simulink model "bObserver"  (R2020a)
settings: Solver=VariableStepAuto  StartTime=0.0  StopTime=1.5  FixedStep=0.0005  EnableMultiTasking=on
InitFcn:
  | kp=0.01;
  | ki=0.01;
  | 
  | k=2;
  | em=100000000;
  | GE=1/em;
  | GU=k*ki/GE;
  | GCE=k*kp/GU;
model workspace (MAT data in the model file):
  time = 0.8
values from neighbouring files (symbols this model uses):
  A1 = obj.boostConverter.A1    [BoostController.m]    (also in BoostConverter.m = [-obj.R/obj.L 0;0 -1/(obj.Ro*obj.C)]; BuckBoostConverter.m = [-obj.R/obj.L 0;0 -1/(obj.Ro*obj.C)]; obsmc.m = Asigma{1,1}; workspace_atual.mat = [-16.4  0; 0  -3.50877192982])
  A2 = obj.boostConverter.A2    [BoostController.m]    (also in BoostConverter.m = [-obj.R/obj.L -1/obj.L;1/obj.C -1/(obj.Ro*obj.C)]; BuckBoostConverter.m = [-obj.R/obj.L 1/obj.L;-1/obj.C -1/(obj.Ro*obj.C)]; obsmc.m = Asigma{1,2}; workspace_atual.mat = [-16.4  -200; 350.877192982  -3.50877192982])
  AlarmDeadTime = 0.50    (= 0.5)    [BoostFaultSimulation.m]    (also in workspace_atual.mat; workspace_certo.mat)
  B1 = obj.boostConverter.B1    [BoostController.m]    (also in BoostConverter.m = [1/obj.L;0]; BuckBoostConverter.m = [1/obj.L;0]; obsmc.m = Bsigma{1,1}; workspace_atual.mat = [200 0])
  B1f = [200 0]    [workspace_atual.mat]    (also in workspace_certo.mat)
  B2 = obj.boostConverter.B2    [BoostController.m]    (also in BoostConverter.m = obj.B1; obsmc.m = Bsigma{1,2}; workspace_atual.mat = [200 0]; workspace_certo.mat = [200 0])
  B2f = [200 0]    [workspace_atual.mat]    (also in workspace_certo.mat)
  boost_Amatrices = cat(3,obj.A1,obj.A2)    [BoostConverter.m]    (also in BuckBoostConverter.m; boostResults2Latex.m = boost.A_matrices(); workspace_atual.mat = [-16.4 0 0 -3.50877192982 -16.4 350.877192982 -200 -3.508771; workspace_certo.mat = [-16.4 0 0 -3.50877192982 -16.4 350.877192982 -200 -3.508771)
  boost_parameters = [obj.Ro,obj.R,obj.L,obj.C,obj.u]'    [BoostConverter.m]    (also in BuckBoostConverter.m; boostResults2Latex.m = boost.parameters(); workspace_atual.mat = [100 0.082 0.005 0.00285 190]; workspace_certo.mat = [100 0.082 0.005 0.00285 190])
  C = 1e-3    (= 0.001)    [boostResults2Latex.m]
  CiL = [0 1]    [workspace_atual.mat]    (also in workspace_certo.mat)
  Cmatrix = [1  0; 0  1]    [workspace_atual.mat]    (also in workspace_certo.mat)
  CVc = [1 0]    [workspace_atual.mat]    (also in workspace_certo.mat)
  D1 = [1  0; 0  1]    [workspace_atual.mat]    (also in workspace_certo.mat)
  F_11 = -16.4    [workspace_atual.mat]    (also in workspace_certo.mat)
  F_12 = -4812476.87956    [workspace_atual.mat]    (also in workspace_certo.mat)
  F_21 = -3.50877192982    [workspace_atual.mat]    (also in workspace_certo.mat)
  F_22 = -2.00703596657    [workspace_atual.mat]    (also in workspace_certo.mat)
  FaultClass = 0    [BoostFaultSimulation.m]    (also in workspace_atual.mat = 1; workspace_certo.mat = 1)
  H_1 = 13715.5123667    [workspace_atual.mat]    (also in workspace_certo.mat)
  iLFaultSwitch = 0    [BoostFaultSimulation.m]    (also in workspace_atual.mat; workspace_certo.mat)
  iLFaultTime = 1.70    (= 1.7)    [BoostFaultSimulation.m]    (also in workspace_atual.mat; workspace_certo.mat)
  iLGainFaultFactor = 15    [BoostFaultSimulation.m]    (also in workspace_atual.mat; workspace_certo.mat)
  iLNoiseFaultSwitch = 0    [BoostFaultSimulation.m]    (also in workspace_atual.mat; workspace_certo.mat)
  iLNoiseTime = 1.70    (= 1.7)    [BoostFaultSimulation.m]    (also in workspace_atual.mat; workspace_certo.mat)
  Jth = 2000    [workspace_atual.mat]    (also in workspace_certo.mat)
  L = 1e-3    (= 0.001)    [boostResults2Latex.m]    (also in obsmc.m = sdpvar(3,1,'full'))
  L_11 = -176809.798019    [workspace_atual.mat]    (also in workspace_certo.mat)
  L_12 = -66005538231.6    [workspace_atual.mat]    (also in workspace_certo.mat)
  L_21 = 0.0967961040176    [workspace_atual.mat]    (also in workspace_certo.mat)
  L_22 = 350.985265141    [workspace_atual.mat]    (also in workspace_certo.mat)
  LoadAddSignalSwitch = 1    [BoostFaultSimulation.m]    (also in workspace_atual.mat; workspace_certo.mat)
  LoadAddSwitch = 0    [BoostFaultSimulation.m]    (also in workspace_atual.mat; workspace_certo.mat)
  LoadAddTime = 0.90    (= 0.9)    [BoostFaultSimulation.m]    (also in workspace_atual.mat; workspace_certo.mat)
  LoadRemoveSignalSwitch = 1    [BoostFaultSimulation.m]    (also in workspace_atual.mat; workspace_certo.mat)
  LoadRemoveSwitch = 0    [BoostFaultSimulation.m]    (also in workspace_atual.mat; workspace_certo.mat)
  LoadRemoveTime = 0.90    (= 0.9)    [BoostFaultSimulation.m]    (also in workspace_atual.mat; workspace_certo.mat)
  LobsiL = [1737913.15707 66180.0912281]    [workspace_atual.mat]    (also in workspace_certo.mat)
  LobsVc = [61200 1]    [workspace_atual.mat]    (also in workspace_certo.mat)
  ObsEp = 70    [workspace_atual.mat]    (also in workspace_certo.mat)
  P = value(P)    [BoostController.m]    (also in boostResults2Latex.m = boost.calculateP(); obsmc.m = blkdiag(1/deltaAtilde(1,2),-1/deltaAtilde(2,1),1); workspace_atual.mat = [0.00235275094895  5.25738510027e-05; 5.25738510027e-05  0.0; workspace_certo.mat = [0.00235275094893  5.25738512446e-05; 5.25738512446e-05  0.0)
  Q_1 = [13715.5123667  1; 1  0]    [workspace_atual.mat]    (also in workspace_certo.mat)
  Q_2 = [1  0; 0.00750867981628  1]    [workspace_atual.mat]    (also in workspace_certo.mat)
  R = 0.1    [boostResults2Latex.m]    (also in workspace_atual.mat = 0.082; workspace_certo.mat = 0.082)
  ReconfigSwitch = 0    [BoostFaultSimulation.m]    (also in workspace_atual.mat; workspace_certo.mat)
  ReconfigTime = 1.707    [BoostFaultSimulation.m]    (also in workspace_atual.mat; workspace_certo.mat)
  rho = 5    [workspace_atual.mat]    (also in workspace_certo.mat)
  RMSfrequency = 47.61    [BoostFaultSimulation.m]    (also in workspace_atual.mat; workspace_certo.mat)
  Ro = 100    [BoostFaultSimulation.m]    (also in boostResults2Latex.m = 10; workspace_atual.mat; workspace_certo.mat)
  Smep = 80    [workspace_atual.mat]    (also in workspace_certo.mat)
  SourceAddSignalSwitch = 1    [BoostFaultSimulation.m]    (also in workspace_atual.mat; workspace_certo.mat)
  SourceAddSwitch = 0    [BoostFaultSimulation.m]    (also in workspace_atual.mat; workspace_certo.mat)
  SourceAddTime = 0.90    (= 0.9)    [BoostFaultSimulation.m]    (also in workspace_atual.mat; workspace_certo.mat)
  SourceAddVoltage = obj.SourceAddFactor*obj.u    [BoostFaultSimulation.m]    (also in workspace_atual.mat = 19; workspace_certo.mat = 19)
  SourceRemoveSignalSwitch = 1    [BoostFaultSimulation.m]    (also in workspace_atual.mat; workspace_certo.mat)
  SourceRemoveSwitch = 0    [BoostFaultSimulation.m]    (also in workspace_atual.mat; workspace_certo.mat)
  SourceRemoveTime = 0.90    (= 0.9)    [BoostFaultSimulation.m]    (also in workspace_atual.mat; workspace_certo.mat)
  SourceRemoveVoltage = obj.SourceRemoveFactor*obj.u    [BoostFaultSimulation.m]    (also in workspace_atual.mat = 19; workspace_certo.mat = 19)
  T_1 = [1 -13715.5123667]    [workspace_atual.mat]    (also in workspace_certo.mat)
  T_2 = [-0.00750867981628 1]    [workspace_atual.mat]    (also in workspace_certo.mat)
  ueq = 0.5    [workspace_atual.mat]    (also in workspace_certo.mat)
  uf = 190    [workspace_atual.mat]    (also in workspace_certo.mat)
  VcFaultSwitch = 0    [BoostFaultSimulation.m]    (also in workspace_atual.mat; workspace_certo.mat)
  VcFaultTime = 1.70    (= 1.7)    [BoostFaultSimulation.m]    (also in workspace_atual.mat; workspace_certo.mat)
  VcGainFaultFactor = 15    [BoostFaultSimulation.m]    (also in workspace_atual.mat; workspace_certo.mat)
  VcNoiseFaultSwitch = 0    [BoostFaultSimulation.m]    (also in workspace_atual.mat; workspace_certo.mat)
  VcNoiseTime = 1.70    (= 1.7)    [BoostFaultSimulation.m]    (also in workspace_atual.mat; workspace_certo.mat)
  ve = 380    [BoostFaultSimulation.m]    (also in boostResults2Latex.m = 100; workspace_atual.mat; workspace_certo.mat)
  x_e = [ie;ve]    [BoostConverter.m]    (also in BuckBoostConverter.m)
  xe = obj.boostConverter.equilibriumstate(ve)    [BoostController.m]    (also in workspace_atual.mat = [7.62509288104 380]; workspace_certo.mat = [7.62509288104 380])
undefined symbols (not defined in the file or in its folder): Atilde1, Atilde2, B1u, Ctilde1, Dtilde1, Dtilde2, F, F1, G, G1, MAXnet, MINnet
libraries: neural x36, powerlib x34, dspstat3 x11, PhdLibrary x10, simulink x7, dspmtrx3 x6, powerlib_meascontrol x4, dspmathops x4
(part 1 of 6)
settings Model: SimulationMode=accelerator  Creator=d13go  LastModifiedBy=vitor
settings SolverCC: MaxConsecutiveZCs=10000  ZeroCrossAlgorithm=Adaptive  DecoupledContinuousIntegration=on  MinimalZcImpactIntegration=on
settings DataIOCC: SaveFinalState=on  SaveState=on  LoggingToFile=on
settings OptimizationCC: DefaultParameterBehavior=Inlined  UseDivisionForNetSlopeComputation=on  GainParamInheritBuiltInType=on  UseFloatMulNetSlope=on  InlineInvariantSignals=on  EfficientFloat2IntCast=on  LifeSpan=1
settings DebuggingCC: ReadBeforeWriteMsg=DisableAll  WriteAfterWriteMsg=DisableAll  WriteAfterReadMsg=DisableAll  AlgebraicLoopMsg=error  MaxConsecutiveZCsMsg=warning  MaskedZcDiagnostic=none  IgnoredZcDiagnostic=none  MultiTaskDSMMsg=none  SFUnexpectedBacktrackingDiag=warning  SFNoUnconditionalDefaultTransitionDiag=warning  ArithmeticOperatorsInVariantConditions=warning
settings HardwareCC: ProdLongLongMode=on
settings ModelReferenceCC: UpdateModelReferenceTargets=IfOutOfDate
settings SFSimCC: SFSimEcho=off  SimUseLocalCustomCode=off  MATLABDynamicMemAlloc=off  CustomCodeUndefinedFunction=UseInterfaceOnly
settings RTWCC: GenerateReport=on  RTWUseLocalCustomCode=off  LaunchReport=on
settings CodeAppCC: ForceParamTrailComments=on
settings GRTTargetCC: TargetLangStandard=C89/C90 (ANSI)  CombineSignalStateStructs=on  MatFileLogging=off  SupportVariableSizeSignals=on
settings ConfigComp: CovMetricSettings=dw  CovHtmlReporting=on  CovSaveCumulativeToWorkspaceVar=on  CovSaveSingleToWorkspaceVar=on  CovExternalEMLEnable=off
settings SimscapeCC: SimscapeNormalizeSystem=off

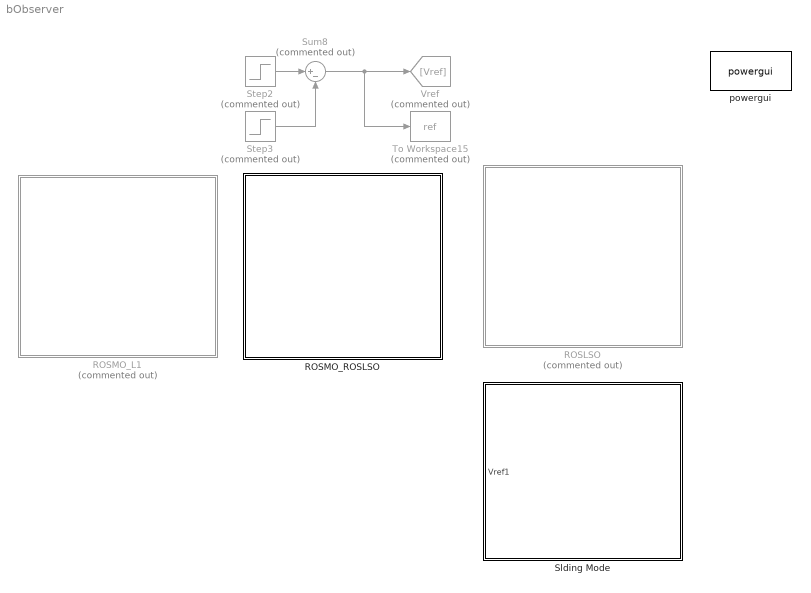
== system bObserver ==
  ROSLSO : Subsystem  Commented=on
  ROSMO_L1 : Subsystem  Commented=on
  ROSMO_ROSLSO : Subsystem
  Slding Mode : Subsystem
  Step2 : Step  Commented=on  Time=0  After=100  SampleTime=0
  Step3 : Step  Commented=on  Time=0.4  After=20  SampleTime=0
  Sum8 : Sum  Commented=on  Inputs=|+-
  To Workspace15 : ToWorkspace  Commented=on  VariableName=ref  SampleTime=-1
  Vref : Goto  Commented=on  GotoTag=Vref
  powergui : powerlib/powergui  Priority=1  SimulationMode=Discrete  SampleTime=50e-6  frequency=60  Iterations=50  frequencyindice=0  Pbase=100e6  ErrMax=1e-4  UnitsV=kV  UnitsW=MW  buscounter=0  FunctionMessages=off  echomessages=off  EnableUseOfTLC=off  CurrentSourceSwitches=off  DisableSnubberDevices=off  DisableRonSwitches=off  DisableVfSwitches=off  DisplayEquations=off  AutomaticDiscreteSolvers=off  SolverType=Tustin/Backward Euler (TBE)  Interpol=off  ExternalGateDelay=off  methode=off  Ts=100  x0status=blocks  SPID=on  SwTol=0  HookPort=off  NonlinearTolerance=1e-4  nMaxIteration=100  ContinueOnMaxIteration=off  RestoreLinks=warning  ResistiveCurrentMeasurement=off  Frange=[0:2:500]  Ylog=off  Xlog=on  ShowGrid=off  save=off  variable=ZData  structure=0  ZoomFFT=off  StartTime=0.0  cycles=1  DisplayStyle=1  fundamental=60  FreqAxis=off  MaxFrequency=1000  frequencyindicesteady=1  RmsSteady=1  display=off
  wires:
  Step2/1 -> Sum8/1
  Step3/1 -> Sum8/2
  Sum8/1 -> To Workspace15/1, Vref/1

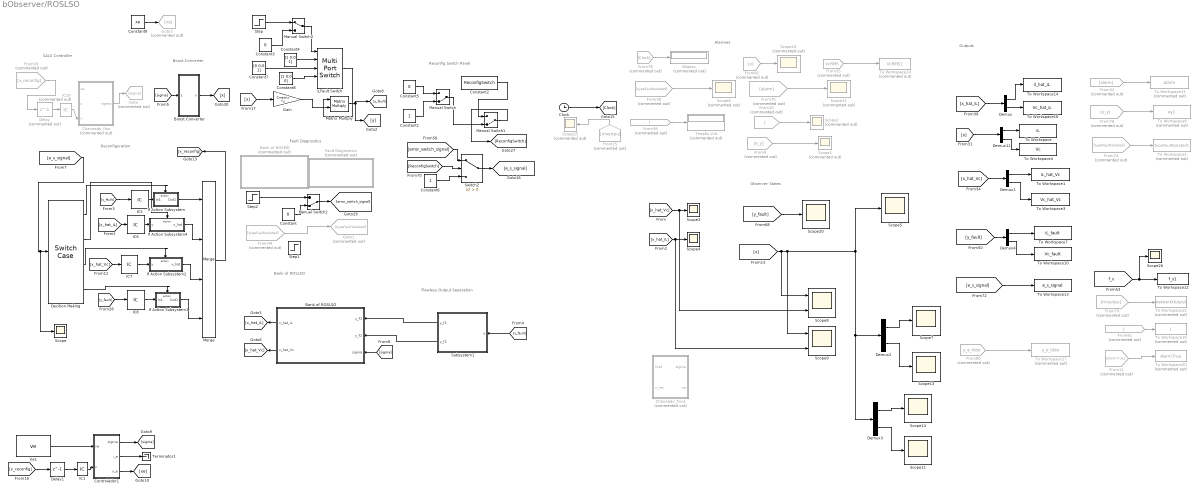
== system bObserver/ROSLSO ==
  note: Fault Diagnostics
  note: Bank of ROSLSO
  note: Reconfiguration
  note: SALS Controller
  note: Boost Converter
  note: Reconfig Switch Panel
  note: Observer States
  note: Outputs
  note: Alarmes
  note: Flawless Output Separation
  Bank of ROSLSO : Subsystem
  Bank of ROSMO : Subsystem  Commented=on
  Boost Converter : Subsystem
  Chaveado_fixo : Subsystem  Commented=on  mask(Switched linear affine Controler){A1=0, A2=0, B1=0, B2=0, P=0}
      mask prompts: A1 "System matrix 1:"; A2 "System matrix 2:"; B1 "Input matrix 1:"; B2 "Input matrix 2:"; P "Gain matrix:"
      mask help: Controller to generate a switching law according to the equilibrium point xe
  Chaveado_fixo1 : Subsystem  Commented=on
  Clock : Clock
  Constant : Constant  Value=0
  Constant1 : Constant
  Constant2 : Constant  Value=ReconfigSwitch
  Constant3 : Constant  Value=0
  Constant4 : Constant  Value=[1 0;0 1]  VectorParams1D=off
  Constant5 : Constant  Value=0
  Constant6 : Constant
  Constant7 : Constant  Value=[0 0;0 1]  VectorParams1D=off
  Constant8 : Constant  Value=[1 0;0 0]  VectorParams1D=off
  Constant9 : Constant  Value=xe
  Controlador1 : Subsystem
  Decition Making : SwitchCase  CaseConditions={[0],[1],[2]}
  Delay : Delay  Commented=on  DelayLength=1
  Delay1 : Delay  DelayLength=1
  Demux{,1..4,11} (6 alike) : Demux  Outputs=2
  Display : Display  Commented=on
  Fault Diagnostics : Subsystem  Commented=on
  From10 : From  Commented=on  GotoTag=J  TagVisibility=global
  From11 : From  Commented=on  GotoTag=alarmTrue
  From15 : From  Commented=on  GotoTag=nnoutpu
  From32 : From  Commented=on  GotoTag=alarm
  From33 : From  Commented=on  GotoTag=x_reconfig
  From35 : From  Commented=on  GotoTag=VcRMS  TagVisibility=global
  From36 : From  Commented=on  GotoTag=J  TagVisibility=global
  From38 : From  Commented=on  GotoTag=typeFaultIsolated
  From44 : From  Commented=on  GotoTag=typeFaultIsolated
  From74 : From  Commented=on  GotoTag=typeFaultIsolated
  From75 : From  Commented=on  GotoTag=alarm
  From76 : From  Commented=on  GotoTag=e_y
  From78 : From  Commented=on  GotoTag=Clock
  From79 : From  Commented=on  GotoTag=nnoutpu
  From80 : From  Commented=on  GotoTag=y_e_tilde  TagVisibility=global
  From81 : From  Commented=on  GotoTag=J  TagVisibility=global
  From82 : From  Commented=on  GotoTag=v
  From9 : From  Commented=on  GotoTag=e_y
  Gain : Gain  Gain=Cmatrix  Multiplication=Matrix(K*u)
  Goto : Goto  Commented=on  GotoTag=sigma
  Goto1 : Goto  Commented=on  GotoTag=typeFaultIsolated
  Goto3 : Goto  Commented=on  GotoTag=xe
  IC{1,5..8} (5 alike) : InitialCondition  Value=[0;0]
  IC10 : InitialCondition  Commented=on  Value=[0;0]
  If Action Subsystem : Subsystem  TreatAsAtomicUnit=on
  If Action Subsystem1 : Subsystem  TreatAsAtomicUnit=on
  If Action Subsystem2 : Subsystem  TreatAsAtomicUnit=on
  If Action Subsystem4 : Subsystem  TreatAsAtomicUnit=on
  Manual Switch : ManualSwitch  CurrentSetting=0
  Manual Switch1 : ManualSwitch  CurrentSetting=0
  Manual Switch2 : ManualSwitch  CurrentSetting=0
  Manual Switch3 : ManualSwitch
  Matrix Multiply : Product  Multiplication=Matrix(*)
  Merge : Merge  Inputs=4
  Scope{,3..5,7,11,13..14,20,26} (10 alike) : Scope
  Scope{1..2,6,10,12,25} (6 alike) : Scope  Commented=on
  Scope8 : Scope  NumInputPorts=2
  Scope9 : Scope  NumInputPorts=2
  Step : Step  Time=0.5  After=2  SampleTime=0
  Step1 : Step  Time=ReconfigTime  Before=1  After=FaultClass  SampleTime=0
  Step2 : Step  Time=0.510  After=2  SampleTime=0
  Subsystem1 : Subsystem
  Switch2 : Switch  Criteria=u2 > Threshold
  Tensão Vc6 : Display  Commented=on
  Terminator1 : Terminator
  To Workspace : ToWorkspace  VariableName=iL  SaveFormat=Timeseries  SampleTime=-1
  To Workspace1 : ToWorkspace  VariableName=iL_hat_Vc  SaveFormat=Timeseries  SampleTime=-1
  To Workspace10 : ToWorkspace  VariableName=Vc_fault  SaveFormat=Timeseries  SampleTime=-1
  To Workspace11 : ToWorkspace  Commented=on  VariableName=Alarm  SaveFormat=Timeseries  SampleTime=-1
  To Workspace12 : ToWorkspace  VariableName=f_s1  SaveFormat=Timeseries  SampleTime=-1
  To Workspace13 : ToWorkspace  VariableName=e_s_signal  SaveFormat=Timeseries  SampleTime=-1
  To Workspace14 : ToWorkspace  VariableName=il_hat_iL  SaveFormat=Timeseries  SampleTime=-1
  To Workspace15 : ToWorkspace  Commented=on  VariableName=networkOutput  SaveFormat=Timeseries  SampleTime=-1
  To Workspace16 : ToWorkspace  VariableName=Vc_hat_iL  SaveFormat=Timeseries  SampleTime=-1
  To Workspace17 : ToWorkspace  Commented=on  VariableName=y_e_tilde  SaveFormat=Timeseries  SampleTime=-1
  To Workspace19 : ToWorkspace  Commented=on  VariableName=J  SaveFormat=Timeseries  SampleTime=-1
  To Workspace2 : ToWorkspace  Commented=on  VariableName=typeFaultIsolated1  SaveFormat=Timeseries  SampleTime=-1
  To Workspace20 : ToWorkspace  Commented=on  VariableName=AlarmTrue  SaveFormat=Timeseries  SampleTime=-1
  To Workspace24 : ToWorkspace  Commented=on  VariableName=VcRMS1  SaveFormat=Timeseries  SampleTime=-1
  To Workspace3 : ToWorkspace  VariableName=Vc_hat_Vc  SaveFormat=Timeseries  SampleTime=-1
  To Workspace4 : ToWorkspace  VariableName=Vc  SaveFormat=Timeseries  SampleTime=-1
  To Workspace7 : ToWorkspace  VariableName=iL_fault  SaveFormat=Timeseries  SampleTime=-1
  To Workspace8 : ToWorkspace  Commented=on  VariableName=ey1  SaveFormat=Timeseries  SampleTime=-1
  Ve1 : Constant  Value=ve
  iLFault Switch : MultiPortSwitch  DataPortOrder=Zero-based contiguous  DataPortForDefault=Additional data port  zeroidx=on
  wires:
  From9/1 -> Scope1/1
  From10/1 -> Scope2/1
  Manual Switch2/1 -> [error_switch_signal]
  Decition Making/1 -> If Action Subsystem/Action
  If Action Subsystem/1(Out1) -> Merge/1
  Decition Making/3 -> If Action Subsystem2/Action
  Clock/1 -> [Clock]
  [ReconfigSwitch] -> Switch2/2
  Manual Switch/1 -> Manual Switch1/2
  Constant1/1 -> Manual Switch/2
  Constant2/1 -> Manual Switch1/1
  Constant5/1 -> Manual Switch/1
  Constant6/1 -> Switch2/3
  Manual Switch1/1 -> [ReconfigSwitch]
  [error_switch_signal] -> Switch2/1
  Decition Making/2 -> If Action Subsystem4/Action
  [y_fault] -> IC8/1
  [x_hat_iL] -> Scope9/2, Scope4/1
  [sigma] -> Boost Converter/1(sigma)
  [x_hat_iL] -> Demux/1
  Demux/1 -> To Workspace14/1
  Demux1/2 -> To Workspace3/1
  From36/1 -> Tensão Vc6/1
  [y_fault] -> Demux4/1
  Demux4/2 -> To Workspace10/1
  From38/1 -> Scope6/1
  From75/1 -> Scope12/1
  From76/1 -> To Workspace8/1
  [f_s] -> Scope26/1, To Workspace12/1
  [y_fault] -> Scope20/1
  From32/1 -> To Workspace11/1
  [e_s_signal] -> To Workspace13/1
  Demux1/1 -> To Workspace1/1
  From74/1 -> To Workspace2/1
  From78/1 -> Display/1
  Demux/2 -> To Workspace16/1
  Demux4/1 -> To Workspace7/1
  [x_hat_Vc] -> Demux1/1
  From79/1 -> To Workspace15/1
  From80/1 -> To Workspace17/1
  From81/1 -> To Workspace19/1
  From82/1 -> Scope10/1
  IC5/1 -> If Action Subsystem/1(In1)
  [y_fault] -> IC5/1
  IC7/1 -> If Action Subsystem2/1(y)
  [x_hat_Vc] -> IC7/1
  IC8/1 -> If Action Subsystem1/1(In1)
  From11/1 -> To Workspace20/1
  Decition Making/4 -> If Action Subsystem1/Action
  IC6/1 -> If Action Subsystem4/1(y)
  If Action Subsystem4/1(x_hat) -> Merge/2
  If Action Subsystem2/1(x_hat) -> Merge/3
  If Action Subsystem1/1(Out1) -> Merge/4
  Merge/1 -> [x_reconfig]
  From15/1 -> Scope25/1
  [x_hat_Vc] -> Scope8/2, Scope3/1
  From35/1 -> To Workspace24/1
  [x] -> Demux11/1
  Demux11/1 -> To Workspace/1
  Demux11/2 -> To Workspace4/1
  [x_hat_iL] -> IC6/1
  [y_fault] -> Subsystem1/1(y)
  Subsystem1/1(y_f1) -> Bank of ROSLSO/1(y_f1)
  Subsystem1/2(y_f2) -> Bank of ROSLSO/2(y_f2)
  [sigma] -> Bank of ROSLSO/3(sigma)
  Bank of ROSLSO/1(x_hat_iL) -> [x_hat_iL]
  Bank of ROSLSO/2(x_hat_Vc) -> [x_hat_Vc]
  [x] -> Scope8/1, Scope9/1, Scope5/1, Demux3/1, Demux2/1
  Switch2/1 -> [e_s_signal]
  IC10/1 -> Chaveado_fixo/3(x)
  Constant9/1 -> Goto3/1
  Chaveado_fixo/1(sigma) -> Goto/1
  [x] -> Gain/1
  Gain/1 -> Matrix Multiply/2
  Matrix Multiply/1 -> [y], [y_fault]
  Constant4/1 -> iLFault Switch/2
  Constant8/1 -> iLFault Switch/4
  Constant7/1 -> iLFault Switch/3
  iLFault Switch/1 -> Matrix Multiply/1
  Boost Converter/1(x) -> [x]
  [e_s_signal] -> Scope/1, Decition Making/1
  Delay/1 -> IC10/1
  From33/1 -> Delay/1
  Step2/1 -> Manual Switch2/1
  Controlador1/3(x_e) -> [xe]
  Controlador1/1(sigma) -> [sigma]
  Controlador1/2(i_e) -> Terminator1/1
  IC1/1 -> Controlador1/2(x)
  [x_reconfig] -> Delay1/1
  Delay1/1 -> IC1/1
  Ve1/1 -> Controlador1/1(ve)
  Demux2/1 -> Scope7/1
  Demux2/2 -> Scope13/1
  Demux3/2 -> Scope11/1
  Demux3/1 -> Scope14/1
  Step/1 -> Manual Switch3/1
  Manual Switch3/1 -> iLFault Switch/1
  Constant3/1 -> Manual Switch3/2
  Constant/1 -> Manual Switch2/2
  From44/1 -> Goto1/1

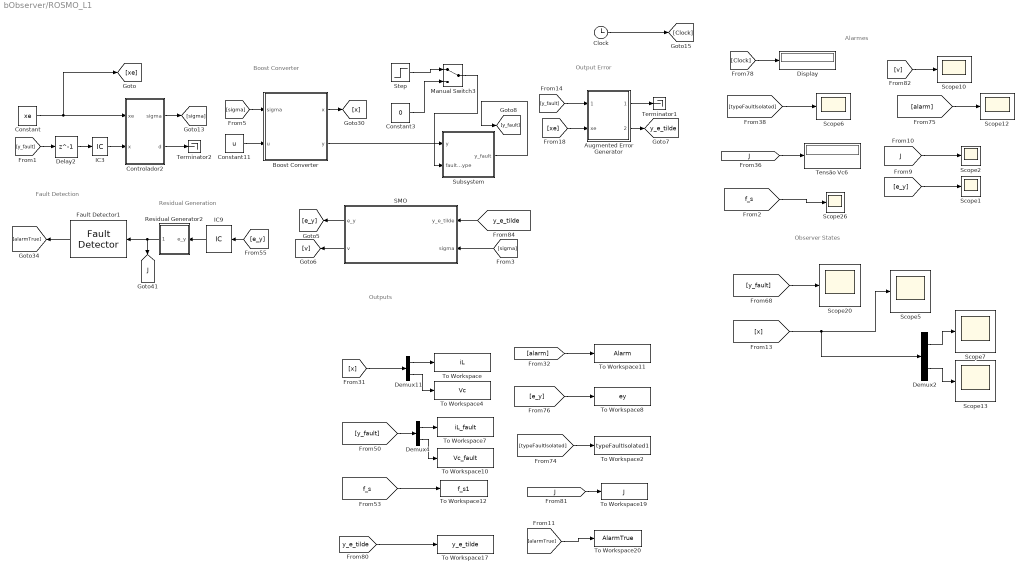
== system bObserver/ROSMO_L1 ==
  note: Boost Converter
  note: Observer States
  note: Outputs
  note: Alarmes
  note: Output Error
  note: Residual Generation
  note: Fault Detection
  Augmented Error Generator : Subsystem  mask{Cmatrix=Cmatrix, Ctilde1=Ctilde1}
      mask prompts: Cmatrix "Output Matrix"; Ctilde1 "Output matrix augmented:"
  Boost Converter : Subsystem  mask(Boots State-Space model){A1=A1, A2=A2, B1=B1, R=R, Ro=Ro, Cmatrix=Cmatrix}
      mask prompts: A1 "A1 matrix"; A2 "A2 matrix"; B1 "B matrix"; R "Resistance"; Ro "Output Resistance"; Cmatrix "Output Matrix"
      mask help: Boots State-Space model
      mask Display: disp('Boost')
  Clock : Clock
  Constant : Constant  Value=xe  VectorParams1D=off
  Constant11 : Constant  Value=u
  Constant3 : Constant  Value=0
  Controlador2 : Subsystem  mask(Sliding mode controller){KiVc=2.3, KVc=0.2, ueq=ueq, Smep=Smep, KiL=2, Freq=7000}
      mask prompts: KiVc "Integral voltage gain"; KVc "Voltage gain"; ueq "Equilibrium signal"; Smep "Surface limit layer"; KiL "Current gain"; Freq "Frequency"
      mask help: Sliding mode controller with integral for boost converter
  Delay2 : Delay  DelayLength=1
  Demux11 : Demux  Outputs=2
  Demux2 : Demux  Outputs=2
  Demux4 : Demux  Outputs=2
  Display : Display
  Fault Detector1 : PhdLibrary/Fault Detector  Jth=0
      settings: SourceProductName=Phd Diego
  IC3 : InitialCondition  Value=[0;0]
  IC9 : InitialCondition  Value=[0;0]
  Manual Switch3 : ManualSwitch
  Residual Generator2 : Subsystem  mask{RMSfrequency=RMSfrequency/10}
      mask prompts: RMSfrequency "Windows length:"
      mask help: RMS generator for two dimensios
  SMO : Subsystem  mask(Sliding mode observer){G=G1, F=F1, Atilde1=Atilde1, Atilde2=Atilde2, Dtilde1=Dtilde1, Dtilde2=Dtilde2, Ctilde1=Ctilde1, rho=rho}
      mask prompts: G "G matrix"; F "F matrix"; Atilde1 "A1 matrix augmented"; Atilde2 "A2 matrix augmented"; Dtilde1 "D1 matrix augmented"; Dtilde2 "D2 matrix augmented"; Ctilde1 "C1 matrix augmented"; rho "Sliding surface coefficient (rho)"
      mask help: Sligin mode observer for fault detection in switched affine linear systems
      mask Help: Enter the system matrices and the observer gains
      mask Display: disp('\dot{x} = Ax + b \\ y = Cx','texmode','on');
  Scope{1..2,5..7,10,12..13,20,26} (10 alike) : Scope
  Step : Step  Time=0.70  SampleTime=0
  Subsystem : Subsystem  mask(Step faults){iLfgain=20, Vcfgain=20}
      mask prompts: iLfgain "Current fault gain (A)"; Vcfgain "Voltage fault gain (V)"
      mask help: Configure a step fault
  Tensão Vc6 : Display
  Terminator1 : Terminator
  Terminator2 : Terminator
  To Workspace : ToWorkspace  VariableName=iL  SaveFormat=Timeseries  SampleTime=-1
  To Workspace10 : ToWorkspace  VariableName=Vc_fault  SaveFormat=Timeseries  SampleTime=-1
  To Workspace11 : ToWorkspace  VariableName=Alarm  SaveFormat=Timeseries  SampleTime=-1
  To Workspace12 : ToWorkspace  VariableName=f_s1  SaveFormat=Timeseries  SampleTime=-1
  To Workspace17 : ToWorkspace  VariableName=y_e_tilde  SaveFormat=Timeseries  SampleTime=-1
  To Workspace19 : ToWorkspace  VariableName=J  SaveFormat=Timeseries  SampleTime=-1
  To Workspace2 : ToWorkspace  VariableName=typeFaultIsolated1  SaveFormat=Timeseries  SampleTime=-1
  To Workspace20 : ToWorkspace  VariableName=AlarmTrue  SaveFormat=Timeseries  SampleTime=-1
  To Workspace4 : ToWorkspace  VariableName=Vc  SaveFormat=Timeseries  SampleTime=-1
  To Workspace7 : ToWorkspace  VariableName=iL_fault  SaveFormat=Timeseries  SampleTime=-1
  To Workspace8 : ToWorkspace  VariableName=ey  SaveFormat=Timeseries  SampleTime=-1
  tag scope: J=global, y_e_tilde=global
  wires:
  [e_y] -> Scope1/1
  [J] -> Scope2/1
  [sigma] -> Boost Converter/1(sigma)
  [J] -> Tensão Vc6/1
  [y_fault] -> Demux4/1
  Demux4/2 -> To Workspace10/1
  [typeFaultIsolated] -> Scope6/1
  [alarm] -> Scope12/1
  [e_y] -> To Workspace8/1
  [f_s] -> To Workspace12/1
  [y_fault] -> Scope20/1
  [alarm] -> To Workspace11/1
  [typeFaultIsolated] -> To Workspace2/1
  [Clock] -> Display/1
  Demux4/1 -> To Workspace7/1
  [y_e_tilde] -> To Workspace17/1
  [J] -> To Workspace19/1
  [v] -> Scope10/1
  [alarmTrue] -> To Workspace20/1
  [x] -> Demux11/1
  Demux11/1 -> To Workspace/1
  Demux11/2 -> To Workspace4/1
  Boost Converter/1(x) -> [x]
  Demux2/1 -> Scope7/1
  Demux2/2 -> Scope13/1
  IC9/1 -> Residual Generator2/1(e_y)
  [e_y] -> IC9/1
  Residual Generator2/1(RMS) -> Fault Detector1/1, [J]
  Controlador2/1(sigma) -> [sigma]
  IC3/1 -> Controlador2/2(x)
  Delay2/1 -> IC3/1
  [y_fault] -> Delay2/1
  SMO/1(e_y) -> [e_y]
  [y_e_tilde] -> SMO/1(y_e_tilde)
  [sigma] -> SMO/2(sigma)
  SMO/2(v) -> [v]
  Constant11/1 -> Boost Converter/2(u)
  Controlador2/2(d) -> Terminator2/1
  Clock/1 -> [Clock]
  Constant/1 -> [xe], Controlador2/1(xe)
  Step/1 -> Manual Switch3/1
  Constant3/1 -> Manual Switch3/2
  Boost Converter/2(y) -> Subsystem/1(y)
  Manual Switch3/1 -> Subsystem/2(faultType)
  Subsystem/1(y_fault) -> [y_fault]
  Augmented Error Generator/2(y_e_tilde) -> [y_e_tilde]
  Augmented Error Generator/1(e_tilde) -> Terminator1/1
  [x] -> Demux2/1, Scope5/1
  [f_s] -> Scope26/1
  [xe] -> Augmented Error Generator/2(xe)
  [y_fault] -> Augmented Error Generator/1(y_fault)
  Fault Detector1/1 -> [alarmTrue]

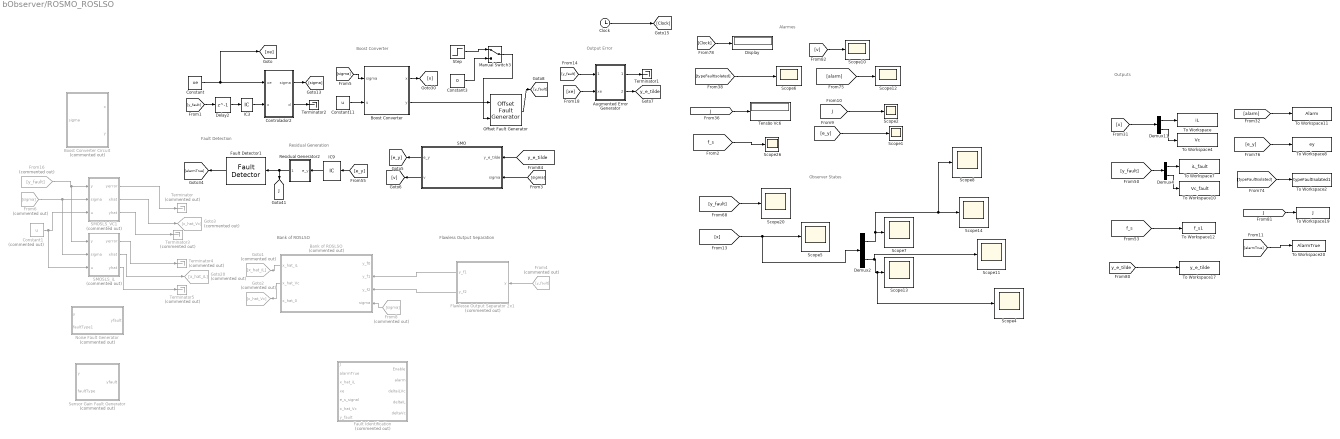
== system bObserver/ROSMO_ROSLSO ==
  note: Boost Converter
  note: Observer States
  note: Outputs
  note: Alarmes
  note: Output Error
  note: Residual Generation
  note: Fault Detection
  note: Bank of ROSLSO
  note: Flawless Output Separation
  Augmented Error Generator : Subsystem  mask{Cmatrix=Cmatrix, Ctilde1=Ctilde1}
      mask prompts: Cmatrix "Output Matrix"; Ctilde1 "Output matrix augmented:"
  Bank of ROSLSO : Subsystem  Commented=on
  Boost Converter : Subsystem  mask(Boots State-Space model){A1=A1, A2=A2, B1=B1, R=R, Ro=Ro, Cmatrix=Cmatrix}
      mask prompts: A1 "A1 matrix"; A2 "A2 matrix"; B1 "B matrix"; R "Resistance"; Ro "Output Resistance"; Cmatrix "Output Matrix"
      mask help: Boots State-Space model
      mask Display: disp('Boost')
  Boost Converter Circuit : Subsystem  Commented=on
  Clock : Clock
  Constant : Constant  Value=xe  VectorParams1D=off
  Constant1 : Constant  Commented=on  Value=u
  Constant11 : Constant  Value=u
  Constant3 : Constant  Value=0
  Controlador2 : Subsystem  mask(Sliding mode controller){KiVc=2.3, KVc=0.2, ueq=ueq, Smep=Smep, KiL=2, Freq=7000}
      mask prompts: KiVc "Integral voltage gain"; KVc "Voltage gain"; ueq "Equilibrium signal"; Smep "Surface limit layer"; KiL "Current gain"; Freq "Frequency"
      mask help: Sliding mode controller with integral for boost converter
  Delay2 : Delay  DelayLength=1
  Demux11 : Demux  Outputs=2
  Demux2 : Demux  Outputs=2
  Demux4 : Demux  Outputs=2
  Display : Display
  Fault Detector1 : PhdLibrary/Fault Detector  Jth=0
      settings: SourceProductName=Phd Diego
  Fault Identification : Subsystem  Commented=on
  Flawlesse Output Separator 2x1 : Subsystem  Commented=on  mask(Flawless Output Separator){Cf1=0, Cf2=0}
      mask prompts: Cf1 "Fault matrix 1"; Cf2 "Fault matrix 2"
      mask help: Separates the 2x1 output
  From16 : From  Commented=on  GotoTag=y_fault  TagVisibility=global
  From4 : From  Commented=on  GotoTag=y_fault
  From6 : From  Commented=on  GotoTag=sigma
  From8 : From  Commented=on  GotoTag=sigma
  Goto1 : Goto  Commented=on  GotoTag=x_hat_iL
  Goto2 : Goto  Commented=on  GotoTag=x_hat_Vc
  Goto20 : Goto  Commented=on  GotoTag=x_hat_iL
  Goto3 : Goto  Commented=on  GotoTag=x_hat_Vc
  IC3 : InitialCondition  Value=[0;0]
  IC9 : InitialCondition  Value=[0;0]
  Manual Switch3 : ManualSwitch
  Noise Fault Generator : Subsystem  Commented=on  mask(Noise fault generator){}
      mask help: Generates noise in the desired sensor
  Offset Fault Generator : PhdLibrary/Offset Fault Generator  s1gain=20  s2gain=20
      settings: SourceProductName=Phd Diego
  Residual Generator2 : Subsystem  mask{RMSfrequency=RMSfrequency/10}
      mask prompts: RMSfrequency "Windows length:"
      mask help: RMS generator for two dimensios
  SMO : Subsystem  mask(Sliding mode observer){G=G1, F=F1, Atilde1=Atilde1, Atilde2=Atilde2, Dtilde1=Dtilde1, Dtilde2=Dtilde2, Ctilde1=Ctilde1, rho=rho}
      mask prompts: G "G matrix"; F "F matrix"; Atilde1 "A1 matrix augmented"; Atilde2 "A2 matrix augmented"; Dtilde1 "D1 matrix augmented"; Dtilde2 "D2 matrix augmented"; Ctilde1 "C1 matrix augmented"; rho "Sliding surface coefficient (rho)"
      mask help: Sligin mode observer for fault detection in switched affine linear systems
      mask Help: Enter the system matrices and the observer gains
      mask Display: disp('\dot{x} = Ax + b \\ y = Cx','texmode','on');
  SMOSLS_VC1 : Subsystem  Commented=on  mask(Sliding mode observer for Switched linear affine systems){A1=A1, A2=A2, B1=B1, B2=B2, C1=CiL, L=LobsiL, Smep=ObsEp, yhat0=0, x0=[0;0]}
      mask prompts: A1 "System matrix 1:"; A2 "System matrix 2:"; B1 "Input matrix 1:"; B2 "Input matrix 2:"; C1 "Output matrix 1:"; L "Observer gain:"; Smep "Limit layer:"; yhat0 "Output initial condition:"; x0 "Observer initial condition:"
      mask help: Full order observer that estimates the full state of a switched affine linear system
  SMOSLS_iL : Subsystem  Commented=on  mask(Sliding mode observer for Switched linear affine systems){A1=A1, A2=A2, B1=B1, B2=B2, C1=CiL, L=LobsiL, Smep=ObsEp, yhat0=0, x0=[0;0]}
      mask prompts: A1 "System matrix 1:"; A2 "System matrix 2:"; B1 "Input matrix 1:"; B2 "Input matrix 2:"; C1 "Output matrix 1:"; L "Observer gain:"; Smep "Limit layer:"; yhat0 "Output initial condition:"; x0 "Observer initial condition:"
      mask help: Full order observer that estimates the full state of a switched affine linear system
  Scope{1..2,4..8,10..14,20,26} (14 alike) : Scope
  Sensor Gain Fault Generator : Subsystem  Commented=on  mask(Sensor gain fault generator){s1gain=0, s2gain=0}
      mask prompts: s1gain "Sensor 1 gain fault:"; s2gain "Sensor 2 gain fault:"
      mask help: Generates a gain fault in each sensor
  Step : Step  Time=0.70  SampleTime=0
  Tensão Vc6 : Display
  Terminator{,3..5} (4 alike) : Terminator  Commented=on
  Terminator1 : Terminator
  Terminator2 : Terminator
  To Workspace : ToWorkspace  VariableName=iL  SaveFormat=Timeseries  SampleTime=-1
  To Workspace10 : ToWorkspace  VariableName=Vc_fault  SaveFormat=Timeseries  SampleTime=-1
  To Workspace11 : ToWorkspace  VariableName=Alarm  SaveFormat=Timeseries  SampleTime=-1
  To Workspace12 : ToWorkspace  VariableName=f_s1  SaveFormat=Timeseries  SampleTime=-1
  To Workspace17 : ToWorkspace  VariableName=y_e_tilde  SaveFormat=Timeseries  SampleTime=-1
  To Workspace19 : ToWorkspace  VariableName=J  SaveFormat=Timeseries  SampleTime=-1
  To Workspace2 : ToWorkspace  VariableName=typeFaultIsolated1  SaveFormat=Timeseries  SampleTime=-1
  To Workspace20 : ToWorkspace  VariableName=AlarmTrue  SaveFormat=Timeseries  SampleTime=-1
  To Workspace4 : ToWorkspace  VariableName=Vc  SaveFormat=Timeseries  SampleTime=-1
  To Workspace7 : ToWorkspace  VariableName=iL_fault  SaveFormat=Timeseries  SampleTime=-1
  To Workspace8 : ToWorkspace  VariableName=ey  SaveFormat=Timeseries  SampleTime=-1
  tag scope: J=global, y_e_tilde=global
  wires:
  [e_y] -> Scope1/1
  [J] -> Scope2/1
  [sigma] -> Boost Converter/1(sigma)
  [J] -> Tensão Vc6/1
  [y_fault] -> Demux4/1
  Demux4/2 -> To Workspace10/1
  [typeFaultIsolated] -> Scope6/1
  [alarm] -> Scope12/1
  [e_y] -> To Workspace8/1
  [f_s] -> To Workspace12/1
  [y_fault] -> Scope20/1
  [alarm] -> To Workspace11/1
  [typeFaultIsolated] -> To Workspace2/1
  [Clock] -> Display/1
  Demux4/1 -> To Workspace7/1
  [y_e_tilde] -> To Workspace17/1
  [J] -> To Workspace19/1
  [v] -> Scope10/1
  [alarmTrue] -> To Workspace20/1
  [x] -> Demux11/1
  Demux11/1 -> To Workspace/1
  Demux11/2 -> To Workspace4/1
  Boost Converter/1(x) -> [x]
  Demux2/1 -> Scope8/1, Scope14/1, Scope7/1
  Demux2/2 -> Scope11/1, Scope4/1, Scope13/1
  IC9/1 -> Residual Generator2/1(e_y)
  [e_y] -> IC9/1
  Residual Generator2/1(RMS) -> Fault Detector1/1, [J]
  Controlador2/1(sigma) -> [sigma]
  IC3/1 -> Controlador2/2(x)
  Delay2/1 -> IC3/1
  [y_fault] -> Delay2/1
  SMO/1(e_y) -> [e_y]
  [y_e_tilde] -> SMO/1(y_e_tilde)
  [sigma] -> SMO/2(sigma)
  SMO/2(v) -> [v]
  Constant11/1 -> Boost Converter/2(u)
  Controlador2/2(d) -> Terminator2/1
  Clock/1 -> [Clock]
  Constant/1 -> [xe], Controlador2/1(xe)
  Step/1 -> Manual Switch3/1
  Constant3/1 -> Manual Switch3/2
  Boost Converter/2(y) -> Offset Fault Generator/1
  Manual Switch3/1 -> Offset Fault Generator/2
  Offset Fault Generator/1 -> [y_fault]
  Augmented Error Generator/2(y_e_tilde) -> [y_e_tilde]
  Augmented Error Generator/1(e_tilde) -> Terminator1/1
  [x] -> Demux2/1, Scope5/1
  [f_s] -> Scope26/1
  [xe] -> Augmented Error Generator/2(xe)
  [y_fault] -> Augmented Error Generator/1(y_fault)
  Flawlesse Output Separator 2x1/2(y_f2) -> Bank of ROSLSO/3(y_f2)
  Bank of ROSLSO/2(x_hat_Vc) -> Goto2/1
  Flawlesse Output Separator 2x1/1(y_f1) -> Bank of ROSLSO/2(y_f1)
  From8/1 -> Bank of ROSLSO/4(sigma)
  From4/1 -> Flawlesse Output Separator 2x1/1(y)
  Bank of ROSLSO/1(x_hat_iL) -> Goto1/1
  Fault Detector1/1 -> [alarmTrue]
  From16/1 -> SMOSLS_iL/1(y), SMOSLS_VC1/1(y)
  From6/1 -> SMOSLS_iL/2(sigma), SMOSLS_VC1/2(sigma)
  Constant1/1 -> SMOSLS_iL/3(u), SMOSLS_VC1/3(u)
  SMOSLS_iL/2(xhat) -> Goto20/1
  SMOSLS_VC1/2(xhat) -> Goto3/1
  SMOSLS_VC1/1(yerror) -> Terminator/1
  SMOSLS_VC1/3(yhat) -> Terminator3/1
  SMOSLS_iL/1(yerror) -> Terminator4/1
  SMOSLS_iL/3(yhat) -> Terminator5/1

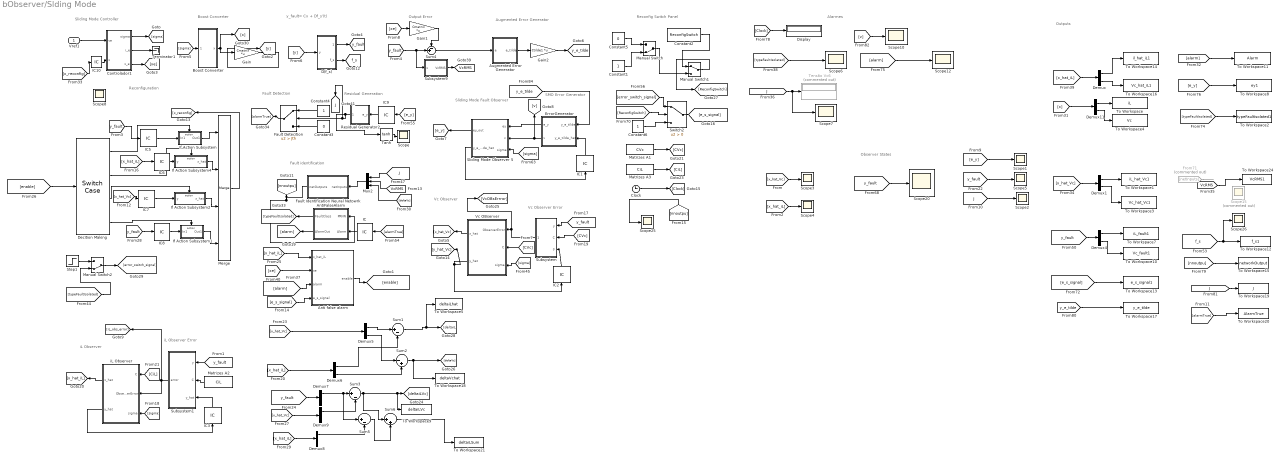
== system bObserver/Slding Mode ==
  note: Reconfiguration
  note: Sliding Mode Controller
  note: Boost Converter
  note: Vc Observer
  note: y_fault= Cx + Df_s'(t)
  note: Output Error
  note: Augmented Error Generator
  note: Sliding Mode
      | Fault Observer
  note: SMO Error
      | Generator
  note: Residual Generation
  note: Fault identification
  note: Reconfig Switch Panel
  note: iL Observer
  note: Vc Observer Error
  note: iL Observer Error
  note: Observer States
  note: Outputs
  note: Alarmes
  note: Fault Detection
  Vref1 : Inport
  Anti false alarm : Subsystem
  AntiFalseAlarm : Subsystem
  Augmented Error Generator : Subsystem
  Boost Converter : Subsystem
  Clock : Clock
  Constant1 : Constant
  Constant2 : Constant  Value=ReconfigSwitch
  Constant3 : Constant  Value=0
  Constant4 : Constant
  Constant5 : Constant  Value=0
  Constant6 : Constant
  Controlador1 : Subsystem
  D(f_s) : Subsystem
  Decition Making : SwitchCase  CaseConditions={[1,6],[2,3],[4,5]}
  Demux{,1,4..9,11} (9 alike) : Demux  Outputs=2
  Display : Display
  ErrorGenerator : Subsystem
  Fault Detecition : Switch  Criteria=u2 > Threshold  Threshold=Jth  ZeroCross=off
  Fault Identification Neural Netowrk : Subsystem
  From71 : From  Commented=on  GotoTag=netInputs  TagVisibility=global
  Gain : Gain  Gain=Cmatrix  Multiplication=Matrix(K*u)
  Gain1 : Gain  Gain=Cmatrix  Multiplication=Matrix(K*u)
  Gain2 : Gain  Gain=Ctilde1  Multiplication=Matrix(K*u)
  IC : InitialCondition  Value=0
  IC{1,5..10} (7 alike) : InitialCondition  Value=[0;0]
  IC2 : InitialCondition  Value=0
  IC3 : InitialCondition  Value=0
  If Action Subsystem : Subsystem  TreatAsAtomicUnit=on
  If Action Subsystem1 : Subsystem  TreatAsAtomicUnit=on
  If Action Subsystem2 : Subsystem  TreatAsAtomicUnit=on
  If Action Subsystem4 : Subsystem  TreatAsAtomicUnit=on
  Manual Switch : ManualSwitch  CurrentSetting=0
  Manual Switch1 : ManualSwitch
  Manual Switch2 : ManualSwitch  CurrentSetting=0
  Matrizes A1 : Constant  Value=CVc  VectorParams1D=off
  Matrizes A2 : Constant  Value=CiL  VectorParams1D=off
  Matrizes A3 : Constant  Value=CiL  VectorParams1D=off
  Merge : Merge  Inputs=4
  Mux2 : Mux  Inputs=3
  Residual Generator2 : Subsystem
  Scope{,1..8,10,12,20,25..26} (14 alike) : Scope
  Scope15 : Scope  Commented=on
  Sliding Mode Observer 5 : Subsystem
  Step1 : Step  Time=ReconfigTime  Before=1  After=FaultClass  SampleTime=0
  Subsystem : Subsystem
  Subsystem1 : Subsystem
  Subsystem9 : Subsystem
  Sum1 : Sum  Inputs=|+-
  Sum2 : Sum  Inputs=|-+
  Sum3 : Sum  Inputs=|+-
  Sum4 : Sum  Inputs=-+|
  Sum5 : Sum  Inputs=|+-
  Sum6 : Sum  Inputs=|++
  Switch2 : Switch  Criteria=u2 > Threshold
  Tanh : Trigonometry  Operator=tanh
  Tensão Vc6 : Display  Commented=on
  Terminator1 : Terminator
  To Workspace : ToWorkspace  VariableName=iL  SaveFormat=Timeseries  SampleTime=-1
  To Workspace1 : ToWorkspace  VariableName=iL_hat_Vc1  SaveFormat=Timeseries  SampleTime=-1
  To Workspace10 : ToWorkspace  VariableName=Vc_fault1  SaveFormat=Timeseries  SampleTime=-1
  To Workspace11 : ToWorkspace  VariableName=Alarm  SaveFormat=Timeseries  SampleTime=-1
  To Workspace12 : ToWorkspace  VariableName=f_s1  SaveFormat=Timeseries  SampleTime=-1
  To Workspace13 : ToWorkspace  VariableName=e_s_signal1  SaveFormat=Timeseries  SampleTime=-1
  To Workspace14 : ToWorkspace  VariableName=il_hat_iL1  SaveFormat=Timeseries  SampleTime=-1
  To Workspace15 : ToWorkspace  VariableName=networkOutput  SaveFormat=Timeseries  SampleTime=-1
  To Workspace16 : ToWorkspace  VariableName=Vc_hat_iL1  SaveFormat=Timeseries  SampleTime=-1
  To Workspace17 : ToWorkspace  VariableName=y_e_tilde  SaveFormat=Timeseries  SampleTime=-1
  To Workspace18 : ToWorkspace  VariableName=deltaVchat  SaveFormat=Timeseries  SampleTime=-1
  To Workspace19 : ToWorkspace  VariableName=J  SaveFormat=Timeseries  SampleTime=-1
  To Workspace2 : ToWorkspace  VariableName=typeFaultIsolated1  SaveFormat=Timeseries  SampleTime=-1
  To Workspace20 : ToWorkspace  VariableName=AlarmTrue  SaveFormat=Timeseries  SampleTime=-1
  To Workspace21 : ToWorkspace  VariableName=deltaiLSum  SaveFormat=Timeseries  SampleTime=-1
  To Workspace24 : ToWorkspace  VariableName=VcRMS1  SaveFormat=Timeseries  SampleTime=-1
  To Workspace3 : ToWorkspace  VariableName=Vc_hat_Vc1  SaveFormat=Timeseries  SampleTime=-1
  To Workspace4 : ToWorkspace  VariableName=Vc  SaveFormat=Timeseries  SampleTime=-1
  To Workspace5 : ToWorkspace  VariableName=deltaiLhat  SaveFormat=Timeseries  SampleTime=-1
  To Workspace7 : ToWorkspace  VariableName=iL_fault1  SaveFormat=Timeseries  SampleTime=-1
  To Workspace8 : ToWorkspace  VariableName=ey1  SaveFormat=Timeseries  SampleTime=-1
  To Workspace9 : ToWorkspace  VariableName=deltaiLVc  SaveFormat=Timeseries  SampleTime=-1
  Vc OBserver : Subsystem
  iL Observer : Subsystem
  tag scope: J=global, VcRMS=global, f_s=global, y_e_tilde=global, y_fault=global
  wires:
  Controlador1/2(i_e) -> Terminator1/1
  Vref1/1 -> Controlador1/1(ve)
  Controlador1/3(x_e) -> [xe]
  Controlador1/1(sigma) -> [sigma]
  Boost Converter/1(x) -> [x], Gain/1
  [sigma] -> Vc OBserver/3(sigma)
  D(f_s)/1(y_fault) -> [y_fault]
  Sum4/1 -> Augmented Error Generator/1(e)
  Augmented Error Generator/1(e_tilde) -> Gain2/1
  [y_e_tilde] -> ErrorGenerator/1(y_e_tilde)
  [e_y] -> Scope1/1
  Gain2/1 -> [y_e_tilde]
  [J] -> Scope2/1
  Mux2/1 -> Fault Identification Neural Netowrk/1(netInputs)
  [J] -> Mux2/1
  Subsystem9/1(VcRMS) -> [VcRMS]
  [typeFaultIsolated] -> Manual Switch2/2
  Manual Switch2/1 -> [error_switch_signal]
  Decition Making/1 -> If Action Subsystem/Action
  If Action Subsystem/1(Out1) -> Merge/1
  Decition Making/3 -> If Action Subsystem2/Action
  [y_fault] -> Subsystem/1(y)
  Clock/1 -> [Clock]
  [ReconfigSwitch] -> Switch2/2
  Switch2/1 -> [e_s_signal]
  Manual Switch/1 -> Manual Switch1/2
  Constant1/1 -> Manual Switch/2
  Constant2/1 -> Manual Switch1/1
  Constant5/1 -> Manual Switch/1
  Constant6/1 -> Switch2/3
  Manual Switch1/1 -> [ReconfigSwitch]
  [error_switch_signal] -> Switch2/1
  Decition Making/2 -> If Action Subsystem4/Action
  Matrizes A2/1 -> Subsystem1/2(C)
  iL Observer/1(x_hat) -> [x_hat_iL]
  Matrizes A1/1 -> [CVc]
  [CVc] -> Subsystem/2(C)
  Matrizes A3/1 -> [CiL]
  [CiL] -> iL Observer/1(C)
  [y_fault] -> IC8/1
  Step1/1 -> Manual Switch2/1
  [x_hat_iL] -> Scope4/1
  [y_fault] -> Scope5/1
  [sigma] -> Boost Converter/1(sigma)
  [alarmTrue] -> IC/1
  AntiFalseAlarm/1(FaultClass) -> [typeFaultIsolated]
  [x_hat_iL] -> Demux/1
  Demux/1 -> To Workspace14/1
  Demux1/2 -> To Workspace3/1
  [J] -> Tensão Vc6/1, Scope7/1
  [y_fault] -> Demux4/1
  Demux4/2 -> To Workspace10/1
  [typeFaultIsolated] -> Scope6/1
  [alarm] -> Scope12/1
  [e_y] -> To Workspace8/1
  [f_s] -> Scope26/1, To Workspace12/1
  [y_fault] -> Scope20/1
  [alarm] -> To Workspace11/1
  [e_s_signal] -> To Workspace13/1
  Demux1/1 -> To Workspace1/1
  From71/1 -> ?
  [typeFaultIsolated] -> To Workspace2/1
  [Clock] -> Display/1
  Demux/2 -> To Workspace16/1
  Demux4/1 -> To Workspace7/1
  [x_hat_Vc] -> Demux1/1
  [nnoutpu] -> To Workspace15/1
  [y_e_tilde] -> To Workspace17/1
  [J] -> To Workspace19/1
  Constant4/1 -> Fault Detecition/1
  Constant3/1 -> Fault Detecition/3
  Fault Detecition/1 -> [alarmTrue]
  [v] -> Scope10/1
  [y_fault] -> Subsystem1/1(y)
  Vc OBserver/2(y_hat) -> IC2/1, [y_hat_Vc]
  [y_fault] -> Subsystem9/1(x), Sum4/2
  Gain/1 -> [y]
  [y] -> D(f_s)/1(y)
  [xe] -> Gain1/1
  Gain1/1 -> Sum4/1
  ErrorGenerator/1(e_y) -> Sliding Mode Observer 5/1(ey)
  ErrorGenerator/2(v) -> Sliding Mode Observer 5/2(v), [v]
  [sigma] -> Sliding Mode Observer 5/3(sigma)
  Sliding Mode Observer 5/2(y_e_tilde_hat) -> IC1/1
  Sliding Mode Observer 5/1(ey_out) -> [e_y]
  IC/1 -> AntiFalseAlarm/2(Alarm)
  Subsystem/1(error) -> [VcOBsErrror], Vc OBserver/1(ObserverError)
  Vc OBserver/1(x_hat) -> [x_hat_Vc]
  [sigma] -> iL Observer/3(sigma)
  Subsystem1/1(error) -> iL Observer/2(ObserverError), [iL_obs_error]
  [CVc] -> Vc OBserver/2(C)
  iL Observer/2(y_hat) -> IC3/1
  IC1/1 -> ErrorGenerator/2(y_e_tilde_hat)
  IC2/1 -> Subsystem/3(y_hat)
  IC3/1 -> Subsystem1/3(y_hat)
  IC5/1 -> If Action Subsystem/1(In1)
  [y_fault] -> IC5/1
  IC7/1 -> If Action Subsystem2/1(y)
  [x_hat_Vc] -> IC7/1
  IC8/1 -> If Action Subsystem1/1(In1)
  [e_y] -> IC9/1
  IC9/1 -> Residual Generator2/1(e_y)
  [x_reconfig] -> IC10/1
  IC10/1 -> Controlador1/2(x)
  AntiFalseAlarm/2(AlarmOut) -> [alarm]
  [alarmTrue] -> To Workspace20/1
  Decition Making/4 -> If Action Subsystem1/Action
  IC6/1 -> If Action Subsystem4/1(y)
  If Action Subsystem4/1(x_hat) -> Merge/2
  [x_hat_Vc] -> Demux5/1
  [x_hat_iL] -> Demux6/1
  Demux5/1 -> Sum1/1
  Demux6/1 -> Sum1/2
  Demux5/2 -> Sum2/1
  Demux6/2 -> Sum2/2
  Sum2/1 -> To Workspace18/1, [deltaVc]
  Fault Identification Neural Netowrk/1(netOutputs) -> AntiFalseAlarm/1(PRNN), [nnoutpu]
  Sum1/1 -> To Workspace5/1, [deltaiL]
  If Action Subsystem2/1(x_hat) -> Merge/3
  If Action Subsystem1/1(Out1) -> Merge/4
  Merge/1 -> [x_reconfig]
  [y_fault] -> Demux7/1
  Demux7/1 -> Sum5/1, Sum3/1
  [x_hat_Vc] -> Demux9/1
  [x_hat_iL] -> Demux8/1
  Demux9/1 -> Sum3/2
  Demux8/1 -> Sum5/2
  [nnoutpu] -> Scope25/1
  [x_hat_Vc] -> Scope3/1
  Sum3/1 -> To Workspace9/1, [deltaiLVc], Sum6/1
  Sum5/1 -> Sum6/2
  Sum6/1 -> To Workspace21/1
  [VcRMS] -> To Workspace24/1
  [VcRMS] -> Mux2/2
  [deltaVc] -> Mux2/3
  Residual Generator2/1(RMS) -> Tanh/1, Fault Detecition/2, [J]
  Tanh/1 -> Scope/1
  [x] -> Demux11/1
  Demux11/1 -> To Workspace/1
  Demux11/2 -> To Workspace4/1
  D(f_s)/2(f_s) -> [f_s]
  [x_hat_iL] -> IC6/1
  [enable] -> Decition Making/1
  [x_hat_iL] -> Anti false alarm/1(x_hat_iL)
  [e_s_signal] -> Anti false alarm/4(e_s_signal)
  [alarm] -> Anti false alarm/3(alarm)
  Anti false alarm/1(enable) -> [enable]
  [xe] -> Anti false alarm/2(xe)

== system bObserver/ROSLSO/Bank of ROSLSO ==
  note: Vc Observer
  note: iL Observer
  y_f1 : Inport
  y_f2 : Inport  Port=2
  sigma : Inport  Port=3
  Constant : Constant  Value=xe  VectorParams1D=off
  Constant1 : Constant  Value=Q_2  VectorParams1D=off
  Constant2 : Constant  Value=T_1  VectorParams1D=off
  Constant8 : Constant  Value=Q_1  VectorParams1D=off
  Matrix Multiply : Product  Multiplication=Matrix(*)
  Matrix Multiply1 : Product  Multiplication=Matrix(*)
  Matrix Multiply2 : Product  Multiplication=Matrix(*)
  Mux : Mux  Inputs=2
  Mux1 : Mux  Inputs=2
  Scope : Scope
  Scope1 : Scope
  Sum : Sum  Inputs=|++
  z1 : Subsystem  Commented=on
  z3 : Subsystem
  z4 : Subsystem
  x_hat_iL : Outport
  x_hat_Vc : Outport  Port=2
  wires:
  sigma/1 -> [sigma]
  [sigma] -> z3/2(sigma)
  y_f1/1 -> z3/1(y_f1), Mux/1
  Mux/1 -> Matrix Multiply/2
  Constant8/1 -> Matrix Multiply/1
  Matrix Multiply/1 -> x_hat_iL/1
  Mux1/1 -> Matrix Multiply1/2
  Matrix Multiply1/1 -> x_hat_Vc/1
  z4/1(z) -> Scope1/1, Mux1/2
  y_f2/1 -> Scope/1, z4/1(y_f2), Mux1/1
  [sigma] -> z4/2(sigma)
  Constant1/1 -> Matrix Multiply1/1
  Constant2/1 -> Matrix Multiply2/1
  Constant/1 -> Matrix Multiply2/2
  Matrix Multiply2/1 -> Sum/2
  z3/1(z) -> Mux/2

== system bObserver/ROSLSO/Bank of ROSMO ==
  note: Vc Observer
  note: iL Observer
  note: Vc Observer Error
  note: iL Observer Error
  IC2 : InitialCondition  Value=0
  IC3 : InitialCondition  Value=0
  Matrizes A2 : Constant  Value=CiL  VectorParams1D=off
  Subsystem : Subsystem
  Subsystem1 : Subsystem
  Vc OBserver : Subsystem
  iL Observer : Subsystem
  wires:
  [CVc] -> Vc OBserver/2(C)
  IC2/1 -> Subsystem/3(y_hat)
  [CiL] -> iL Observer/1(C)
  [sigma] -> Vc OBserver/3(sigma)
  [y_fault] -> Subsystem1/1(y)
  [y_fault] -> Subsystem/1(y)
  Matrizes A2/1 -> Subsystem1/2(C)
  iL Observer/1(x_hat) -> [x_hat_iL]
  [CVc] -> Subsystem/2(C)
  Vc OBserver/2(y_hat) -> IC2/1, [y_hat_Vc]
  Subsystem/1(error) -> [VcOBsErrror], Vc OBserver/1(ObserverError)
  iL Observer/2(y_hat) -> IC3/1
  [sigma] -> iL Observer/3(sigma)
  Vc OBserver/1(x_hat) -> [x_hat_Vc]
  Subsystem1/1(error) -> iL Observer/2(ObserverError), [iL_obs_error]
  IC3/1 -> Subsystem1/3(y_hat)

== system bObserver/ROSLSO/Boost Converter ==
  sigma : Inport
  Constant2 : Constant  Value=B1*u  VectorParams1D=off
  Constant4 : Constant  Value=A1  VectorParams1D=off
  Constant5 : Constant  Value=A2  VectorParams1D=off
  Integral : Subsystem
  Matrix Multiply : Product  Multiplication=Matrix(*)
  Matrix Multiply2 : Product  Multiplication=Matrix(*)
  Sum : Sum  Inputs=|++
  Sum1 : Sum  Inputs=|++
  Switch1 : Switch  Criteria=u2 ~= 0
  x : Outport
  wires:
  [A1x] -> Sum/1
  Constant2/1 -> [Bu]
  [x] -> Matrix Multiply2/2, Matrix Multiply/2
  [Bu] -> Sum1/2
  [Bu] -> Sum/2
  Constant5/1 -> Matrix Multiply2/1
  Constant4/1 -> Matrix Multiply/1
  Matrix Multiply2/1 -> [A2x]
  [sys1] -> Switch1/1
  Matrix Multiply/1 -> [A1x]
  Sum/1 -> [sys1]
  Sum1/1 -> [sys2]
  [sys2] -> Switch1/3
  Switch1/1 -> Integral/1(x_dot)  "x"
  [A2x] -> Sum1/1
  sigma/1 -> Switch1/2
  Integral/1(x) -> x/1, [x]

== system bObserver/ROSLSO/Chaveado_fixo ==
  xe : Inport
  u : Inport  Port=2
  x : Inport  Port=3
  Constant1 : Constant  Value=A1  VectorParams1D=off
  Constant2 : Constant  Value=P  VectorParams1D=off
  Constant3 : Constant  Value=B1  VectorParams1D=off
  Constant4 : Constant
  Constant5 : Constant  Value=A2  VectorParams1D=off
  Constant6 : Constant  Value=0
  Constant8 : Constant  Value=B2  VectorParams1D=off
  Matrix Multiply{1..4} (4 alike) : Product  Multiplication=Matrix(*)
  Sum : Sum  Inputs=|+-
  Sum1 : Sum  Inputs=|+-
  Sum2 : Sum  Inputs=|+-
  Sum3 : Sum  Inputs=|++
  Switch1 : Switch  Criteria=u2 > Threshold
  Transpose : Math  Operator=transpose  SaturateOnIntegerOverflow=on
  sigma : Outport
  wires:
  Constant5/1 -> Sum2/2
  Matrix Multiply2/1 -> Switch1/2
  [control_matrix] -> Transpose/1
  Constant1/1 -> Sum2/1
  Constant6/1 -> Switch1/1
  Sum/1 -> Matrix Multiply2/2
  [xe] -> Sum/2
  [x] -> Sum/1
  Constant4/1 -> Switch1/3
  x/1 -> [x]
  Transpose/1 -> Matrix Multiply2/1
  Constant2/1 -> Matrix Multiply3/1
  Switch1/1 -> sigma/1  "z"
  Constant3/1 -> Sum1/1
  Constant8/1 -> Sum1/2
  Sum2/1 -> Matrix Multiply1/1
  Sum1/1 -> Matrix Multiply4/1
  u/1 -> Matrix Multiply4/2
  xe/1 -> [xe], Matrix Multiply1/2
  Matrix Multiply1/1 -> Sum3/1
  Matrix Multiply4/1 -> Sum3/2
  Sum3/1 -> Matrix Multiply3/2
  Matrix Multiply3/1 -> [control_matrix]

== system bObserver/ROSLSO/Chaveado_fixo1 ==
  note: Controlador
  Vref : Inport
  x_rec : Inport  Port=2
  Controlador Chavead : Subsystem
  sigma : Outport
  xe : Outport  Port=2
  wires:
  Vref/1 -> [Vref], Controlador Chavead/1(Ve)
  Controlador Chavead/3(i_e) -> [iref]
  x_rec/1 -> Controlador Chavead/2(x)
  Controlador Chavead/1(sigma) -> sigma/1
  Controlador Chavead/2(x_e) -> xe/1
